simulink library "WZM_QSS_Lib"  (Simulink 7.7)
settings: Solver=ode45  StartTime=0.0  StopTime=10.0  RelTol=1e-3
undefined symbols (not defined in the file): A, AirCompressor, CNC, Housing, HydraulicPump, MainDrive, MainDriveCoolingEx, Process, ProcessCooling, R
libraries: WZM_QSS_Lib x36
(part 1 of 2)
settings Model: Creator=simon  LastModifiedBy=Coni

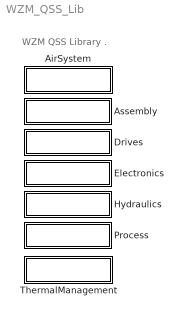
== system WZM_QSS_Lib ==
  note: WZM QSS Library
      | .
  AirSystem : Subsystem
      mask Display: disp('Air System')
  Assembly : Subsystem
      mask Display: disp('Assembly')
  Drives : Subsystem
      mask Display: disp('Drives')
  Electronics : Subsystem
      mask Display: disp('Electronics')
  Hydraulics : Subsystem
      mask Display: disp('Hydraulics')
  Process : Subsystem
      mask Display: disp('Process')
  ThermalManagement : Subsystem
      mask Display: disp('Thermal\nManagement')

== system WZM_QSS_Lib/AirSystem ==
  AirCompressor : Subsystem  BlockChoice=AirCompressor_Dummy
      settings: TemplateBlock=self  MemberBlocks=AirCompressor_Dummy,AirCompressor_Simple
  AirCompressor_Dummy : Subsystem
  AirCompressor_Simple : Subsystem  mask{Pstandby=0, Pworking=0}
      mask prompts: Pstandby "Standby consumption [W]"; Pworking "Working consumption [W]"

== system WZM_QSS_Lib/Assembly ==
  Turning Machine : Subsystem  mask{MainDrive=MainDrive, MainDriveCoolingEx=MainDriveCoolingEx, CNC=CNC, Process=Process, ProcessCooling=ProcessCooling, Housing=Housing, AirCompressor=AirCompressor, HydraulicPump=HydraulicPump, LocMainDrive=machine housing, LocProcessCooling=shop floor, LocProcess=process housing, LocMachine=shop floor, LocMachineExtr=shop floor, LocCNC=shop floor, LocCNCExtr=shop floor, LocAirCompressor=shop floor, LocHydraulicPump=shop floor}
      mask prompts: MainDrive "Main drive parameters"; MainDriveCoolingEx "Main drive cooling parameters"; CNC "CNC cabinet parameters"; Process "Process parameters"; ProcessCooling "Process cooling Parameters"; Housing "Housing Parameters"; AirCompressor "Air compressor Parameters"; HydraulicPump "Hydraulic pump Parameters"; LocMainDrive "Main drive cooling heat flow to"; LocProcessCooling "Process cooling heat flow to"; LocProcess "Process heat flow to"; LocMachine "Machine convective heat flow to"; LocMachineExtr "Machine cooling heat flow to"; LocCNC "Cabinet convective heat flow to"; LocCNCExtr "Cabinet cooling heat flow to"; LocAirCompressor "Air compressor heat flow to"; LocHydraulicPump "Hydraulic pump heat flow to"
      mask help:
      | Simple turning machine with:
      | - Air cooled process
      | - Air cooled machine housing
      | - Air-ar cooled cabinet
      mask StyleString: edit,edit,edit,edit,edit,edit,edit,edit,popup(process housing|machine housing|shop floor|external cooling),popup(process housing|machine housing|shop floor|external cooling),popup(process housing|machine housing|shop floor|external cooling),popup(process housing|machine housing|shop floor|external cooling),popup(process housing|machine housing|shop floor|external cooling),popup(process housing|machine housing|shop floor|external cooling),popup(process housing|machine housing|shop floor|external cooling),popup(process housing|machine housing|shop floor|external cooling),popup(process housing|machine housing|shop floor|external cooling)
      mask TabNameString: Parameters,Parameters,Parameters,Parameters,Parameters,Parameters,Parameters,Parameters,Heat management,Heat management,Heat management,Heat management,Heat management,Heat management,Heat management,Heat management,Heat management

== system WZM_QSS_Lib/Drives ==
  MainDrive : Subsystem  BlockChoice=MainDrive_simple
      settings: TemplateBlock=self  MemberBlocks=MainDrive_Dummy,MainDrive_simple
  MainDrive_Dummy : Subsystem  mask{P_max=20e3, eta=0.92, theta=1}
      mask prompts: P_max "Maximal mechanical power [W]"; eta "Efficiency of the motor [1]"; theta "Momentum of inertia of the drive [kg m^2]"
      mask help: Maps a demanded rotational speed and torque to the corresponding energy demand, heat generation and avaiable mechanical power.
      mask Display: disp('MAIN DRIVE');
  MainDrive_simple : Subsystem  mask{P_max=20e3, eta=0.92, theta=1, Tomega=MainDrive.Tabelomega, TM=MainDrive.TabelM, Teta=MainDrive.Tabeleta}
      mask prompts: P_max "Maximal mechanical power [W]"; eta "Efficiency of the motor [1]"; theta "Momentum of inertia of the drive [kg m^2]"; Tomega "Tabel omega"; TM "Tabel M"; Teta "Teabel eta"
      mask help: Maps a demanded rotational speed and torque to the corresponding energy demand, heat generation and avaiable mechanical power.
      mask Display: disp('MAIN DRIVE');
  Motor : Subsystem  mask{Pmax=10000, eta=.9, g=on}
      mask prompts: Pmax "Maximal absolute mechanical power [W]"; eta "Efficiency [1]"; g "Generator mode possible"
      mask help: Simple motor model. Maps the input u=P_dem/P_max to the produced mechanical power, the generated heat and the demanded electrical power.

== system WZM_QSS_Lib/Electronics ==
  CNC_Cabinet : Subsystem  BlockChoice=CNC_Cabinet_AirCooledFan_ao
      settings: TemplateBlock=self  MemberBlocks=CNC_Cabinet_AirAirCooled_Hyst,CNC_Cabinet_AirCooledFan_ao
  CNC_Cabinet_AirAirCooled_Hyst : Subsystem  mask{Cabinet=0, Cooling=0, SimoDrive=0}
      mask prompts: Cabinet "Cabinet Parameters"; Cooling "Air-air-cooling Parameters"; SimoDrive "Simodrive Parameters"
      mask help:
      | Parameters:
      |
      | - Cabinet.m
      | - Cabinet.cp
      | - Cabinet.R
      | - Cabinet.A
      |
      | - SimoDrive.OpPointsP
      | - SimoDrive.OpPointsEta
      | - SimoDrive.PStandby
      |
      | - Cooling.T_int
      | - Cooling.T_ext
      | - Cooling.Qdot
      | - Cooling.Tmin
      | - Cooling.Tmax
  CNC_Cabinet_AirCooledFan_ao : Subsystem  mask{Cabinet=0, Fan=0, SimoDrive=0}
      mask prompts: Cabinet "Cabinet Parameters"; Fan "Fan Parameters"; SimoDrive "Simodrive Parameters"
      mask help:
      | Parameters:
      |
      | - Cabinet.m
      | - Cabinet.cp
      | - Cabinet.R
      | - Cabinet.A
      |
      | - SimoDrive.OpPointsP
      | - SimoDrive.OpPointsEta
      | - SimoDrive.PStandby
      |
      | - Fan.Vdotnom
      | - Fan.Pnom
  Simodrive : Subsystem  mask{OpPointsP=0, OpPointsEta=0, Pstandby=0, g=off}
      mask prompts: OpPointsP "Operation points [W]"; OpPointsEta "Corresponding efficiencies [-]"; Pstandby "Standby consumption [W]"; g "Enable negative power"
      mask init:
      | if g==1
      |     g=-inf;
      | end

== system WZM_QSS_Lib/Hydraulics ==
  HydraulicPump : Subsystem  BlockChoice=HydraulicPump_Dummy
      settings: TemplateBlock=self  MemberBlocks=HydraulicPump_Dummy,HydraulicPump_Simple
  HydraulicPump_Dummy : Subsystem
  HydraulicPump_Simple : Subsystem  mask{Pconst=0}
      mask prompts: Pconst "Power consumption when running [W]"

== system WZM_QSS_Lib/Process ==
  ProcessModel : Subsystem  BlockChoice=Process_simple
      settings: TemplateBlock=self  MemberBlocks=Process_dummy,Process_simple
  Process_dummy : Subsystem
  Process_simple : Subsystem  mask{eta=0}
      mask prompts: eta "Efficiency of the process [1]"
      mask help: Simple process model: Mechanical work is converted to process work with constant efficiency

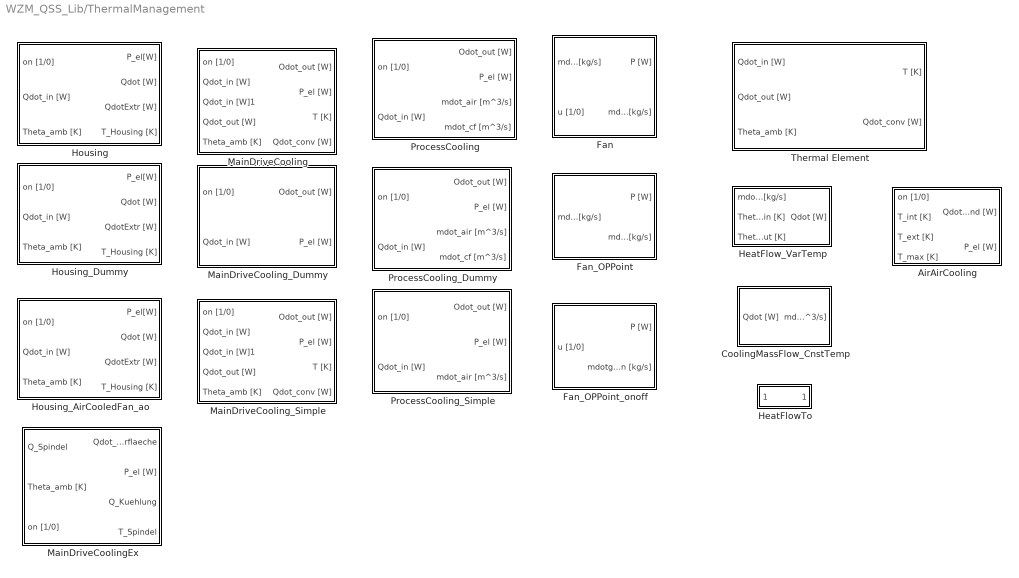
== system WZM_QSS_Lib/ThermalManagement ==
  AirAirCooling : Subsystem  mask{T_int_Pnts=0, T_amb_Pnts=0, Qdot_extr_Pnts=0, epsilon=0}
      mask prompts: T_int_Pnts "Internal temperature operation points [K]"; T_amb_Pnts "External temperature operation points [K]"; Qdot_extr_Pnts "Corresponding heat flow f(T_int,T_ext) [W]"; epsilon "COP of the cooling element"
  CoolingMassFlow_CnstTemp : Subsystem  mask{cp=0, Tin=0, Tout=0}
      mask prompts: cp "Internal heat capacity of the medium [J/kg/k]"; Tin "Inlet temperature [K]"; Tout "Outlet temperature [K]"
  Fan : Subsystem  BlockChoice=Fan_OPPoint
      settings: TemplateBlock=self  MemberBlocks=Fan_OPPoint,Fan_OPPoint_onoff
  Fan_OPPoint : Subsystem  mask{Vdotnom=1, Pnom=1, rho=1.2}
      mask prompts: Vdotnom "Nominal troughput [m^3/s]"; Pnom "Nominal electrical power consumption [W]"; rho "Desity of the  [kg/m^3]"
      mask help:
      | Simple model of a ventilator. Given a nominal operation point:
      | P = Pnom*(Vdem/Vnom)^3
      settings: AttributesFormatString=Vdotnom = %<Vdotnom> m^3/s\nPnom = %<Pnom> W\nDesity = %<rho> kg/m^3
      mask Display:
      | a = 0:.1:2*pi;
      | plot(.5+.3*cos(a),.5+.3*sin(a))
      | a1 = pi/6;
      | a2 = pi/2+pi/6;
      | x = .5+.3*[cos(a1), cos(a2)];
      | y = .5+.3*[sin(a1), sin(a2)];
      | plot(x,y)
      | plot(x([2 1]),y-.4)
  Fan_OPPoint_onoff : Subsystem  mask{Vdotnom=1, Pnom=1, rho=1.2}
      mask prompts: Vdotnom "Nominal troughput [m^3/s]"; Pnom "Nominal electrical power consumption [W]"; rho "Desity of the  [kg/m^3]"
      mask help:
      | Simple model of a ventilator. Given a nominal operation point:
      | P = Pnom*(Vdem/Vnom)^3
      settings: AttributesFormatString=Vdotnom = %<Vdotnom> m^3/s\nPnom = %<Pnom> W\nDesity = %<rho> kg/m^3
      mask Display:
      | a = 0:.1:2*pi;
      | plot(.5+.3*cos(a),.5+.3*sin(a))
      | a1 = pi/6;
      | a2 = pi/2+pi/6;
      | x = .5+.3*[cos(a1), cos(a2)];
      | y = .5+.3*[sin(a1), sin(a2)];
      | plot(x,y)
      | plot(x([2 1]),y-.4)
  HeatFlowTo : Subsystem  mask{Loc=process housing, LocNum=0}
      mask prompts: Loc "Heat flow to"; LocNum "Heat flow to 1=process housing, 2=machine housing, 3=shop floor, 4=external cooling (Keep zero while using popup above)]"
      mask help: Defines where the heat flux is going to
      mask init:
      | if LocNum ~=0
      |     Loc = LocNum;
      | end
      | 
      | idx = zeros(4,1);
      | idx(Loc)=1;
      settings: AttributesFormatString=%<Loc>
      mask StyleString: popup(process housing|machine housing|shop floor|external cooling),edit
      mask TabNameString: Popup,Numeric
      mask Display:
      | plot([0 1],[0.5 .9])
      | plot([0 1],[0.5 .6])
      | plot([0 1],[0.5 .4])
      | plot([0 1],[0.5 .1])
      | plot([1 1],[1 0])
  HeatFlow_VarTemp : Subsystem  mask{cp=1200}
      mask prompts: cp "Internal heat capacity of the medium [J/kg/k]"
  Housing : Subsystem  BlockChoice=Housing_AirCooledFan_ao
      settings: TemplateBlock=self  MemberBlocks=Housing_AirCooledFan_ao,Housing_Dummy
  Housing_AirCooledFan_ao : Subsystem  mask{Cabinet=0, Fan=0}
      mask prompts: Cabinet "Housing Parameters"; Fan "Fan Parameters"
      mask help:
      | Parameters:
      |
      | - Cabinet.m
      | - Cabinet.cp
      | - Cabinet.R
      | - Cabinet.A
      |
      | - Fan.Vdotnom
      | - Fan.Pnom
  Housing_Dummy : Subsystem
  MainDriveCooling : Subsystem  BlockChoice=MainDriveCooling_Dummy
      settings: TemplateBlock=self  MemberBlocks=MainDriveCooling_Dummy,MainDriveCooling_Simple
  MainDriveCoolingEx : Subsystem  mask{Temperatur=MainDriveCoolingEx.Temperatur, AirCooling=MainDriveCoolingEx.Air, TController=MainDriveCoolingEx}
      mask prompts: Temperatur "Tempeatur"; TController "TemperaturController"
  MainDriveCooling_Dummy : Subsystem
  MainDriveCooling_Simple : Subsystem  mask{OpPointQ=0, OpPointEpsilon=0, Pon=0}
      mask prompts: OpPointQ "Operation point heat flow"; OpPointEpsilon "Corresponding cooling index"; Pon "Idle consumption [W]"
  ProcessCooling : Subsystem  BlockChoice=ProcessCooling_Dummy
      settings: TemplateBlock=self  MemberBlocks=ProcessCooling_Dummy,ProcessCooling_Simple
  ProcessCooling_Dummy : Subsystem
  ProcessCooling_Simple : Subsystem  mask{Pconst=0}
      mask prompts: Pconst "Constant power demand [W]"
  Thermal Element : Subsystem  mask{m=10, cp=1200, R=0, A=2}
      mask prompts: m "Internal mass [kg]"; cp "Internal heat capacity [J/kg/K]"; R "Heat transfer resistance of the surface [W/m^2/K]"; A "Surface area [m^2]"
      mask help: Simple

== system WZM_QSS_Lib/AirSystem/AirCompressor ==
  on [1/0] : Inport
  mdot [kg/s] : Inport  Port=2
  AirCompressor_Dummy : WZM_QSS_Lib/AirSystem/AirCompressor_Dummy  SystemSampleTime=-1
  P_el [W] : Outport
  Qdot [W] : Outport  Port=2
  wires:
  on [1/0]/1 -> AirCompressor_Dummy/1
  mdot [kg/s]/1 -> AirCompressor_Dummy/2
  AirCompressor_Dummy/1 -> P_el [W]/1
  AirCompressor_Dummy/2 -> Qdot [W]/1

== system WZM_QSS_Lib/AirSystem/AirCompressor_Dummy ==
  on [1/0] : Inport
  mdot [kg/s] : Inport  Port=2
  Constant : Constant  Value=0
  Constant1 : Constant  Value=0
  Terminator : Terminator
  Terminator1 : Terminator
  P_el [W] : Outport
  Qdot [W] : Outport  Port=2
  wires:
  Constant/1 -> P_el [W]/1
  Constant1/1 -> Qdot [W]/1
  on [1/0]/1 -> Terminator/1
  mdot [kg/s]/1 -> Terminator1/1

== system WZM_QSS_Lib/AirSystem/AirCompressor_Simple ==
  on [1/0] : Inport
  mdot [kg/s] : Inport  Port=2
  Constant : Constant  Value=0
  Constant1 : Constant  Value=Pstandby
  Constant2 : Constant  Value=Pworking
  Switch : Switch  Criteria=u2 > Threshold
  Switch1 : Switch  Criteria=u2 > Threshold
  P_el [W] : Outport
  wires:
  Switch/1 -> P_el [W]/1
  on [1/0]/1 -> Switch/2
  mdot [kg/s]/1 -> Switch1/2
  Switch1/1 -> Switch/1
  Constant2/1 -> Switch1/1
  Constant/1 -> Switch1/3
  Constant1/1 -> Switch/3

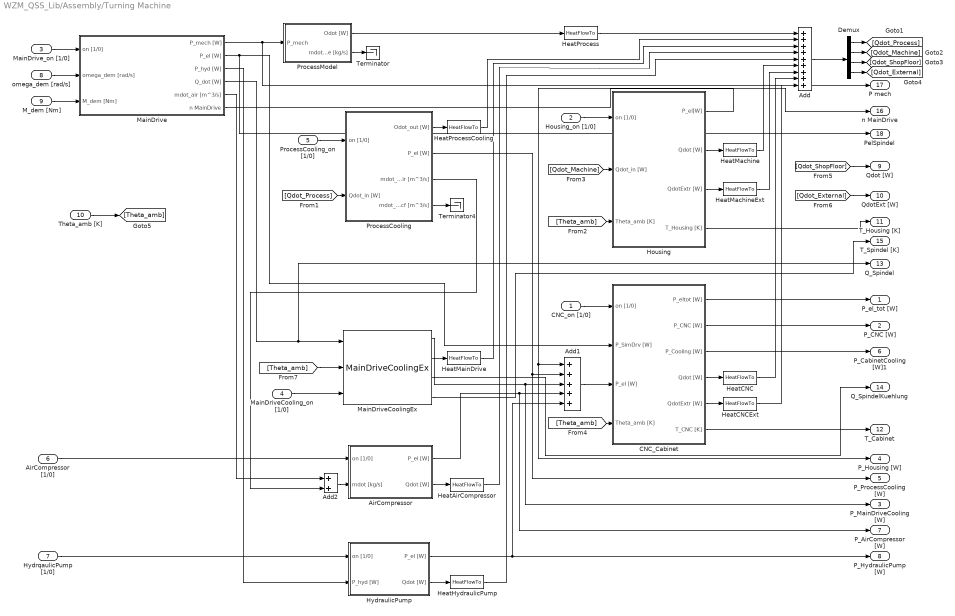
== system WZM_QSS_Lib/Assembly/Turning Machine ==
  CNC_on [1/0] : Inport
  Housing_on [1/0] : Inport  Port=2
  MainDrive_on [1/0] : Inport  Port=3
  MainDriveCooling_on [1/0] : Inport  Port=4
  ProcessCooling_on [1/0] : Inport  Port=5
  AirCompressor [1/0] : Inport  Port=6
  HydrqaulicPump [1/0] : Inport  Port=7
  omega_dem [rad/s] : Inport  Port=8
  M_dem [Nm] : Inport  Port=9
  Theta_amb [K] : Inport  Port=10
  Add : Sum  Inputs=+++++++++
  Add1 : Sum  Inputs=+++++
  Add2 : Sum
  AirCompressor : Subsystem  BlockChoice=AirCompressor_Simple
      link override AirCompressor_Simple: Pstandby=AirCompressor.Pstandby  Pworking=AirCompressor.Pworking
      settings: AttributesFormatString=%<BlockChoice>  TemplateBlock=WZM_QSS_Lib/AirSystem/AirCompressor  MemberBlocks=AirCompressor_Dummy,AirCompressor_Simple
  CNC_Cabinet : Subsystem  BlockChoice=CNC_Cabinet_AirAirCooled_Hyst
      link override CNC_Cabinet_AirAirCooled_Hyst: Cabinet=CNC.Cabinet  Cooling=CNC.Cooling  SimoDrive=CNC.SimoDrive
      link override CNC_Cabinet_AirCooledFan_ao: Cabinet=CNC.Cabinet  Fan=CNC.Fan  PstandbySDSimoDrive=CNC.Fan  SimoDrive=CNC.SimoDrive
      settings: AttributesFormatString=%<BlockChoice>  TemplateBlock=WZM_QSS_Lib/Electronics/CNC_Cabinet  MemberBlocks=CNC_Cabinet_AirAirCooled_Hyst,CNC_Cabinet_AirCooledFan_ao
  Demux : Demux
  HeatAirCompressor : WZM_QSS_Lib/ThermalManagement/HeatFlowTo  SystemSampleTime=-1  Loc=machine housing  LocNum=LocAirCompressor
      settings: AttributesFormatString=%<Loc>
  HeatCNC : WZM_QSS_Lib/ThermalManagement/HeatFlowTo  SystemSampleTime=-1  Loc=shop floor  LocNum=LocCNC
      settings: AttributesFormatString=%<Loc>
  HeatCNCExt : WZM_QSS_Lib/ThermalManagement/HeatFlowTo  SystemSampleTime=-1  Loc=shop floor  LocNum=LocCNCExtr
      settings: AttributesFormatString=%<Loc>
  HeatHydraulicPump : WZM_QSS_Lib/ThermalManagement/HeatFlowTo  SystemSampleTime=-1  Loc=machine housing  LocNum=LocHydraulicPump
      settings: AttributesFormatString=%<Loc>
  HeatMachine : WZM_QSS_Lib/ThermalManagement/HeatFlowTo  SystemSampleTime=-1  Loc=shop floor  LocNum=LocMachine
      settings: AttributesFormatString=%<Loc>
  HeatMachineExt : WZM_QSS_Lib/ThermalManagement/HeatFlowTo  SystemSampleTime=-1  Loc=shop floor  LocNum=LocMachineExtr
      settings: AttributesFormatString=%<Loc>
  HeatMainDrive : WZM_QSS_Lib/ThermalManagement/HeatFlowTo  SystemSampleTime=-1  Loc=machine housing  LocNum=LocMainDrive
      settings: AttributesFormatString=%<Loc>
  HeatProcess : WZM_QSS_Lib/ThermalManagement/HeatFlowTo  SystemSampleTime=-1  Loc=process housing  LocNum=LocProcess
      settings: AttributesFormatString=%<Loc>
  HeatProcessCooling : WZM_QSS_Lib/ThermalManagement/HeatFlowTo  SystemSampleTime=-1  Loc=shop floor  LocNum=LocProcessCooling
      settings: AttributesFormatString=%<Loc>
  Housing : Subsystem  BlockChoice=Housing_AirCooledFan_ao
      link override Housing_AirCooledFan_ao: Cabinet=Housing.Cabinet  Fan=Housing.Fan
      settings: AttributesFormatString=%<BlockChoice>  TemplateBlock=WZM_QSS_Lib/ThermalManagement/Housing  MemberBlocks=Housing_AirCooledFan_ao,Housing_Dummy
  HydraulicPump : Subsystem  BlockChoice=HydraulicPump_Simple
      link override HydraulicPump_Simple: Pconst=HydraulicPump.Pconst
      settings: AttributesFormatString=%<BlockChoice>  TemplateBlock=WZM_QSS_Lib/Hydraulics/HydraulicPump  MemberBlocks=HydraulicPump_Dummy,HydraulicPump_Simple
  MainDrive : Subsystem  BlockChoice=MainDrive_simple
      link override MainDrive_simple: P_max=MainDrive.Pmax  eta=MainDrive.eta  theta=MainDrive.Theta
      settings: AttributesFormatString=%<BlockChoice>  TemplateBlock=WZM_QSS_Lib/Drives/MainDrive  MemberBlocks=MainDrive_Dummy,MainDrive_simple
  MainDriveCoolingEx : WZM_QSS_Lib/ThermalManagement/MainDriveCoolingEx  SystemSampleTime=-1  Temperatur=MainDriveCoolingEx.Temperatur  AirCooling=MainDriveCoolingEx.Air  TController=MainDriveCoolingEx
  ProcessCooling : Subsystem  BlockChoice=ProcessCooling_Simple
      link override ProcessCooling_Simple: Pconst=ProcessCooling.Pconst
      settings: AttributesFormatString=%<BlockChoice>  TemplateBlock=WZM_QSS_Lib/ThermalManagement/ProcessCooling  MemberBlocks=ProcessCooling_Dummy,ProcessCooling_Simple
  ProcessModel : Subsystem  BlockChoice=Process_simple
      link override Process_simple: eta=Process.eta
      settings: AttributesFormatString=%<BlockChoice>  TemplateBlock=WZM_QSS_Lib/Process/ProcessModel  MemberBlocks=Process_dummy,Process_simple
  Terminator : Terminator
  Terminator4 : Terminator
  P_el_tot [W] : Outport
  P_CNC [W] : Outport  Port=2
  P_MainDriveCooling [W] : Outport  Port=3
  P_Housing [W] : Outport  Port=4
  P_ProcessCooling [W] : Outport  Port=5
  P_CabinetCooling [W]1 : Outport  Port=6
  P_AirCompressor [W] : Outport  Port=7
  P_HydraulicPump [W] : Outport  Port=8
  Qdot [W] : Outport  Port=9
  QdotExt [W] : Outport  Port=10
  T_Housing [K] : Outport  Port=11
  T_Cabinet : Outport  Port=12
  Q_Spindel : Outport  Port=13
  Q_SpindelKuehlung : Outport  Port=14
  T_Spindel [K] : Outport  Port=15
  n MainDrive : Outport  Port=16
  P mech : Outport  Port=17
  PelSpindel : Outport  Port=18
  wires:
  MainDriveCooling_on [1/0]/1 -> MainDriveCoolingEx/3
  [Theta_amb] -> MainDriveCoolingEx/2
  MainDrive/1(P_mech [W]) -> ProcessModel/1(P_mech), P mech/1
  CNC_Cabinet/1(P_eltot [W]) -> P_el_tot [W]/1
  CNC_on [1/0]/1 -> CNC_Cabinet/1(on [1/0])
  ProcessModel/1(Odot [W]) -> HeatProcess/1
  Add/1 -> Demux/1
  Demux/1 -> [Qdot_Process]
  Demux/2 -> [Qdot_Machine]
  Demux/3 -> [Qdot_ShopFloor]
  Demux/4 -> [Qdot_External]
  HeatProcess/1 -> Add/1
  HeatCNC/1 -> Add/8
  HeatCNCExt/1 -> Add/9
  Housing_on [1/0]/1 -> Housing/1(on [1/0])
  Theta_amb [K]/1 -> [Theta_amb]
  [Theta_amb] -> Housing/3(Theta_amb [K])
  [Qdot_Machine] -> Housing/2(Qdot_in [W])
  [Theta_amb] -> CNC_Cabinet/4(Theta_amb [K])
  Housing/2(Qdot [W]) -> HeatMachine/1
  Housing/3(QdotExtr [W]) -> HeatMachineExt/1
  HeatMachineExt/1 -> Add/7
  HeatMachine/1 -> Add/6
  Add1/1 -> CNC_Cabinet/3(P_el [W])
  Housing/1(P_el[W]) -> Add1/1, P_Housing [W]/1
  [Qdot_ShopFloor] -> Qdot [W]/1
  [Qdot_External] -> QdotExt [W]/1
  Housing/4(T_Housing [K]) -> T_Housing [K]/1
  MainDriveCoolingEx/2 -> Add1/3, P_MainDriveCooling [W]/1
  MainDriveCoolingEx/1 -> HeatMainDrive/1
  ProcessModel/2(mdot_waste [kg/s]) -> Terminator/1
  M_dem [Nm]/1 -> MainDrive/3(M_dem [Nm])
  omega_dem [rad/s]/1 -> MainDrive/2(omega_dem [rad/s])
  MainDrive_on [1/0]/1 -> MainDrive/1(on [1/0])
  ProcessCooling_on [1/0]/1 -> ProcessCooling/1(on [1/0])
  [Qdot_Process] -> ProcessCooling/2(Qdot_in [W])
  MainDrive/3(P_hyd [W]) -> HydraulicPump/2(P_hyd [W])
  MainDrive/2(P_el [W]) -> CNC_Cabinet/2(P_SimDrv [W]), PelSpindel/1
  ProcessCooling/1(Odot_out [W]) -> HeatProcessCooling/1
  HeatMainDrive/1 -> Add/3
  HeatProcessCooling/1 -> Add/2
  ProcessCooling/2(P_el [W]) -> Add1/2, P_ProcessCooling [W]/1
  ProcessCooling/3(mdot_air [m^3/s]) -> Add2/2
  ProcessCooling/4(mdot_cf [m^3/s]) -> Terminator4/1
  MainDrive/4(Q_dot [W]) -> MainDriveCoolingEx/1, Q_Spindel/1
  CNC_Cabinet/2(P_CNC [W]) -> P_CNC [W]/1
  CNC_Cabinet/6(T_CNC [K]) -> T_Cabinet/1
  CNC_Cabinet/5(QdotExtr [W]) -> HeatCNCExt/1
  CNC_Cabinet/4(Qdot [W]) -> HeatCNC/1
  CNC_Cabinet/3(P_Cooling [W]) -> P_CabinetCooling [W]1/1
  AirCompressor/1(P_el [W]) -> Add1/4, P_AirCompressor [W]/1
  AirCompressor/2(Qdot [W]) -> HeatAirCompressor/1
  HeatAirCompressor/1 -> Add/4
  Add2/1 -> AirCompressor/2(mdot [kg/s])
  MainDrive/5(mdot_air [m^3/s]) -> Add2/1
  AirCompressor [1/0]/1 -> AirCompressor/1(on [1/0])
  HydraulicPump/1(P_el [W]) -> Add1/5, P_HydraulicPump [W]/1
  HydrqaulicPump [1/0]/1 -> HydraulicPump/1(on [1/0])
  HydraulicPump/2(Qdot [W]) -> HeatHydraulicPump/1
  HeatHydraulicPump/1 -> Add/5
  MainDriveCoolingEx/3 -> Q_SpindelKuehlung/1
  MainDriveCoolingEx/4 -> T_Spindel [K]/1
  MainDrive/6(n MainDrive) -> n MainDrive/1

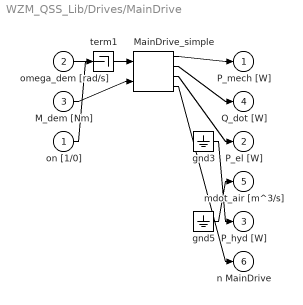
== system WZM_QSS_Lib/Drives/MainDrive ==
  on [1/0] : Inport
  omega_dem [rad/s] : Inport  Port=2
  M_dem [Nm] : Inport  Port=3
  MainDrive_simple : WZM_QSS_Lib/Drives/MainDrive_simple  SystemSampleTime=-1  P_max=20e3  eta=0.92  theta=1  Tomega=MainDrive.Tabelomega  TM=MainDrive.TabelM  Teta=MainDrive.Tabeleta
  gnd3 : Ground
  gnd5 : Ground
  term1 : Terminator
  P_mech [W] : Outport
  P_el [W] : Outport  Port=2
  P_hyd [W] : Outport  Port=3
  Q_dot [W] : Outport  Port=4
  mdot_air [m^3/s] : Outport  Port=5
  n MainDrive : Outport  Port=6
  wires:
  omega_dem [rad/s]/1 -> MainDrive_simple/1
  M_dem [Nm]/1 -> MainDrive_simple/2
  MainDrive_simple/1 -> P_mech [W]/1
  MainDrive_simple/2 -> Q_dot [W]/1
  MainDrive_simple/3 -> P_el [W]/1
  MainDrive_simple/4 -> n MainDrive/1
  on [1/0]/1 -> term1/1
  gnd3/1 -> P_hyd [W]/1
  gnd5/1 -> mdot_air [m^3/s]/1

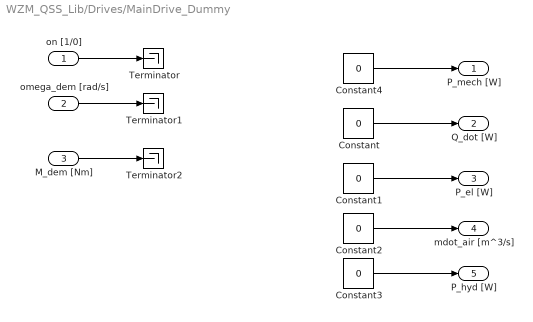
== system WZM_QSS_Lib/Drives/MainDrive_Dummy ==
  on [1/0] : Inport
  omega_dem [rad/s] : Inport  Port=2
  M_dem [Nm] : Inport  Port=3
  Constant{,1..4} (5 alike) : Constant  Value=0
  Terminator : Terminator
  Terminator1 : Terminator
  Terminator2 : Terminator
  P_mech [W] : Outport
  Q_dot [W] : Outport  Port=2
  P_el [W] : Outport  Port=3
  mdot_air [m^3/s] : Outport  Port=4
  P_hyd [W] : Outport  Port=5
  wires:
  on [1/0]/1 -> Terminator/1
  omega_dem [rad/s]/1 -> Terminator1/1
  M_dem [Nm]/1 -> Terminator2/1
  Constant4/1 -> P_mech [W]/1
  Constant/1 -> Q_dot [W]/1
  Constant1/1 -> P_el [W]/1
  Constant2/1 -> mdot_air [m^3/s]/1
  Constant3/1 -> P_hyd [W]/1

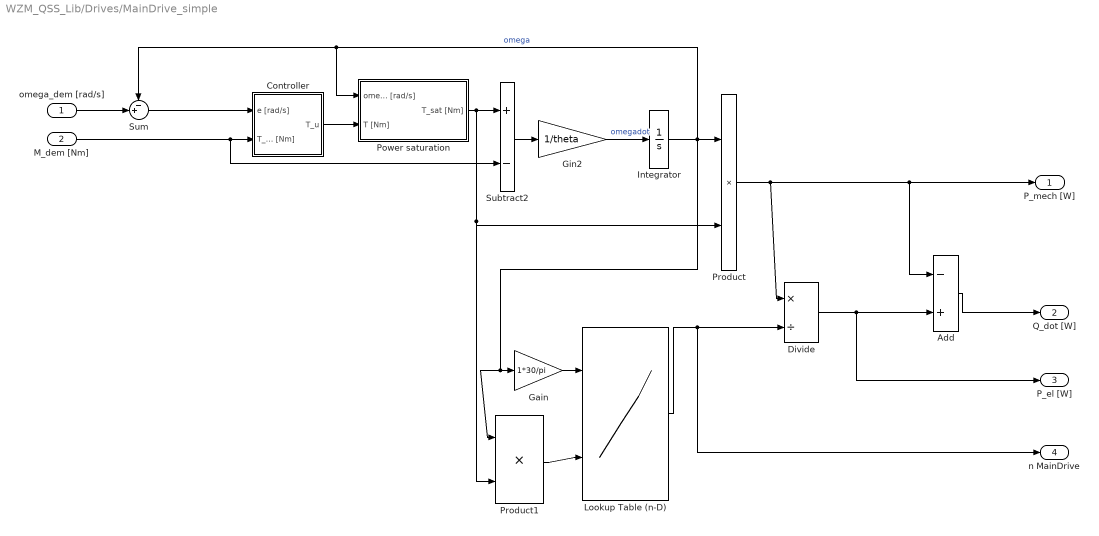
== system WZM_QSS_Lib/Drives/MainDrive_simple ==
  omega_dem [rad/s] : Inport
  M_dem [Nm] : Inport  Port=2
  Add : Sum  Inputs=-+
  Controller : Subsystem
  Divide : Product  Inputs=*/
  Gain : Gain  Gain=1*30/pi
  Gin2 : Gain  Gain=1/theta
  Integrator : Integrator
  Lookup Table (n-D) : Lookup_n-D  BreakpointsForDimension1=Tomega  BreakpointsForDimension2=TM  Table=Teta  InterpMethod=Cubic spline  ExtrapMethod=Cubic spline  InputSameDT=on
  Power saturation : Subsystem
  Product : Product  RndMeth=Zero
  Product1 : Product  RndMeth=Zero
  Subtract2 : Sum  Inputs=+-
  Sum : Sum  Inputs=-+|
  P_mech [W] : Outport
  Q_dot [W] : Outport  Port=2
  P_el [W] : Outport  Port=3
  n MainDrive : Outport  Port=4
  wires:
  Integrator/1 -> Product/1, Sum/1, Power saturation/1(omega [rad/s]), Gain/1, Product1/1  "omega"
  Product/1 -> Divide/1, P_mech [W]/1, Add/1
  Gin2/1 -> Integrator/1  "omegadot"
  omega_dem [rad/s]/1 -> Sum/2
  Sum/1 -> Controller/1(e [rad/s])
  M_dem [Nm]/1 -> Subtract2/2, Controller/2(T_dem [Nm])
  Controller/1(T_u) -> Power saturation/2(T [Nm])
  Subtract2/1 -> Gin2/1
  Power saturation/1(T_sat [Nm]) -> Subtract2/1, Product/2, Product1/2
  Add/1 -> Q_dot [W]/1
  Lookup Table (n-D)/1 -> Divide/2, n MainDrive/1
  Divide/1 -> P_el [W]/1, Add/2
  Gain/1 -> Lookup Table (n-D)/1
  Product1/1 -> Lookup Table (n-D)/2

== system WZM_QSS_Lib/Drives/Motor ==
  u [1] : Inport
  Abs : Abs
  Saturation : Saturate  UpperLimit=1  LowerLimit=-g
  ain : Gain  Gain=Pmax
  ain1 : Gain  Gain=1/eta-1
  ain2 : Gain  Gain=1/eta
  P_mech [W] : Outport
  Qdot [W] : Outport  Port=2
  P_el [W] : Outport  Port=3
  wires:
  u [1]/1 -> Saturation/1
  Saturation/1 -> ain/1
  ain/1 -> P_mech [W]/1, ain2/1, Abs/1
  ain1/1 -> Qdot [W]/1
  ain2/1 -> P_el [W]/1
  Abs/1 -> ain1/1

== system WZM_QSS_Lib/Electronics/CNC_Cabinet ==
  on [1/0] : Inport
  P_SimDrv [W] : Inport  Port=2
  P_el [W] : Inport  Port=3
  Theta_amb [K] : Inport  Port=4
  CNC_Cabinet_AirCooledFan_ao : WZM_QSS_Lib/Electronics/CNC_Cabinet_AirCooledFan_ao  SystemSampleTime=-1  Cabinet=0  Fan=0  SimoDrive=0
  gnd3 : Ground
  P_eltot [W] : Outport
  P_CNC [W] : Outport  Port=2
  P_Cooling [W] : Outport  Port=3
  Qdot [W] : Outport  Port=4
  QdotExtr [W] : Outport  Port=5
  T_CNC [K] : Outport  Port=6
  wires:
  on [1/0]/1 -> CNC_Cabinet_AirCooledFan_ao/1
  P_SimDrv [W]/1 -> CNC_Cabinet_AirCooledFan_ao/2
  P_el [W]/1 -> CNC_Cabinet_AirCooledFan_ao/3
  Theta_amb [K]/1 -> CNC_Cabinet_AirCooledFan_ao/4
  CNC_Cabinet_AirCooledFan_ao/1 -> P_eltot [W]/1
  CNC_Cabinet_AirCooledFan_ao/2 -> P_CNC [W]/1
  CNC_Cabinet_AirCooledFan_ao/3 -> Qdot [W]/1
  CNC_Cabinet_AirCooledFan_ao/4 -> QdotExtr [W]/1
  CNC_Cabinet_AirCooledFan_ao/5 -> T_CNC [K]/1
  gnd3/1 -> P_Cooling [W]/1

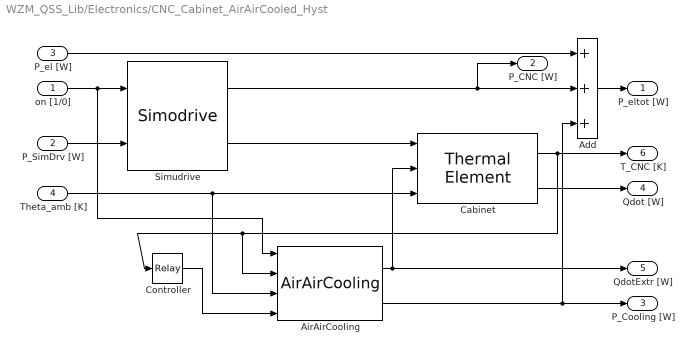
== system WZM_QSS_Lib/Electronics/CNC_Cabinet_AirAirCooled_Hyst ==
  on [1/0] : Inport
  P_SimDrv [W] : Inport  Port=2
  P_el [W] : Inport  Port=3
  Theta_amb [K] : Inport  Port=4
  Add : Sum  Inputs=+++
  AirAirCooling : WZM_QSS_Lib/ThermalManagement/AirAirCooling  SystemSampleTime=-1  T_int_Pnts=Cooling.T_int  T_amb_Pnts=Cooling.T_ext  Qdot_extr_Pnts=Cooling.Qdot  epsilon=Cooling.epsilon
  Cabinet : WZM_QSS_Lib/ThermalManagement/Thermal Element  SystemSampleTime=-1  m=Cabinet.m  cp=Cabinet.cp  R=Cabinet.R  A=Cabinet.A
  Controller : Relay  OnSwitchValue=Cooling.Tmax  OffSwitchValue=Cooling.Tmin
  Simudrive : WZM_QSS_Lib/Electronics/Simodrive  SystemSampleTime=-1  OpPointsP=SimoDrive.OpPointsP  OpPointsEta=SimoDrive.OpPointsEta  Pstandby=SimoDrive.PStandby  g=off
  P_eltot [W] : Outport
  P_CNC [W] : Outport  Port=2
  P_Cooling [W] : Outport  Port=3
  Qdot [W] : Outport  Port=4
  QdotExtr [W] : Outport  Port=5
  T_CNC [K] : Outport  Port=6
  wires:
  on [1/0]/1 -> Simudrive/1, AirAirCooling/1
  Theta_amb [K]/1 -> Cabinet/3, AirAirCooling/3
  Cabinet/1 -> T_CNC [K]/1, Controller/1, AirAirCooling/2
  Add/1 -> P_eltot [W]/1
  Cabinet/2 -> Qdot [W]/1
  P_SimDrv [W]/1 -> Simudrive/2
  Simudrive/2 -> Cabinet/1
  Simudrive/1 -> P_CNC [W]/1, Add/2
  P_el [W]/1 -> Add/1
  AirAirCooling/1 -> QdotExtr [W]/1, Cabinet/2
  AirAirCooling/2 -> Add/3, P_Cooling [W]/1
  Controller/1 -> AirAirCooling/4

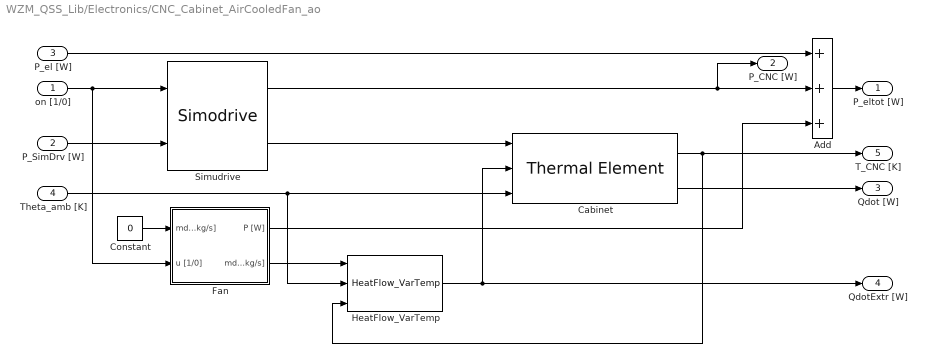
== system WZM_QSS_Lib/Electronics/CNC_Cabinet_AirCooledFan_ao ==
  on [1/0] : Inport
  P_SimDrv [W] : Inport  Port=2
  P_el [W] : Inport  Port=3
  Theta_amb [K] : Inport  Port=4
  Add : Sum  Inputs=+++
  Cabinet : WZM_QSS_Lib/ThermalManagement/Thermal Element  SystemSampleTime=-1  m=Cabinet.m  cp=Cabinet.cp  R=Cabinet.R  A=Cabinet.A
  Constant : Constant  Value=0
  Fan : Subsystem  BlockChoice=Fan_OPPoint_onoff
      link override Fan_OPPoint: Vdotnom=Fan.Vdotnom  Pnom=Fan.Pnom
      settings: AttributesFormatString=%<BlockChoice>  TemplateBlock=WZM_QSS_Lib/ThermalManagement/Fan  MemberBlocks=Fan_OPPoint,Fan_OPPoint_onoff
  HeatFlow_VarTemp : WZM_QSS_Lib/ThermalManagement/HeatFlow_VarTemp  SystemSampleTime=-1  cp=1005
  Simudrive : WZM_QSS_Lib/Electronics/Simodrive  SystemSampleTime=-1  OpPointsP=SimoDrive.OpPointsP  OpPointsEta=SimoDrive.OpPointsEta  Pstandby=SimoDrive.PStandby  g=off
  P_eltot [W] : Outport
  P_CNC [W] : Outport  Port=2
  Qdot [W] : Outport  Port=3
  QdotExtr [W] : Outport  Port=4
  T_CNC [K] : Outport  Port=5
  wires:
  P_el [W]/1 -> Add/1
  Simudrive/1 -> Add/2, P_CNC [W]/1
  Simudrive/2 -> Cabinet/1
  P_SimDrv [W]/1 -> Simudrive/2
  HeatFlow_VarTemp/1 -> QdotExtr [W]/1, Cabinet/2
  Fan/2(mdotgen [kg/s]) -> HeatFlow_VarTemp/1
  Cabinet/2 -> Qdot [W]/1
  Fan/1(P [W]) -> Add/3
  Add/1 -> P_eltot [W]/1
  Cabinet/1 -> HeatFlow_VarTemp/3, T_CNC [K]/1
  Theta_amb [K]/1 -> HeatFlow_VarTemp/2, Cabinet/3
  Constant/1 -> Fan/1(mdot [kg/s])
  on [1/0]/1 -> Simudrive/1, Fan/2(u [1/0])

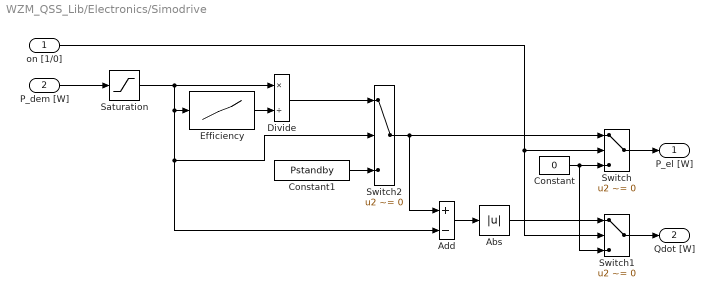
== system WZM_QSS_Lib/Electronics/Simodrive ==
  on [1/0] : Inport
  P_dem [W] : Inport  Port=2
  Abs : Abs
  Add : Sum  Inputs=+-
  Constant : Constant  Value=0
  Constant1 : Constant  Value=Pstandby
  Divide : Product  Inputs=*/
  Efficiency : Lookup_n-D  NumberOfTableDimensions=1  BreakpointsForDimension1=OpPointsP  Table=OpPointsEta  UseLastTableValue=on  RndMeth=Simplest  InputSameDT=on
  Saturation : Saturate  UpperLimit=Inf  LowerLimit=g
  Switch : Switch  Criteria=u2 ~= 0
  Switch1 : Switch  Criteria=u2 ~= 0
  Switch2 : Switch  Criteria=u2 ~= 0
  P_el [W] : Outport
  Qdot [W] : Outport  Port=2
  wires:
  Switch/1 -> P_el [W]/1
  Switch1/1 -> Qdot [W]/1
  Constant/1 -> Switch/3, Switch1/3
  P_dem [W]/1 -> Saturation/1
  Constant1/1 -> Switch2/3
  Efficiency/1 -> Divide/2
  on [1/0]/1 -> Switch1/2, Switch/2
  Add/1 -> Abs/1
  Switch2/1 -> Add/1, Switch/1
  Divide/1 -> Switch2/1
  Abs/1 -> Switch1/1
  Saturation/1 -> Divide/1, Efficiency/1, Switch2/2, Add/2

== system WZM_QSS_Lib/Hydraulics/HydraulicPump ==
  on [1/0] : Inport
  P_hyd [W] : Inport  Port=2
  HydraulicPump_Dummy : WZM_QSS_Lib/Hydraulics/HydraulicPump_Dummy  SystemSampleTime=-1
  P_el [W] : Outport
  Qdot [W] : Outport  Port=2
  wires:
  on [1/0]/1 -> HydraulicPump_Dummy/1
  P_hyd [W]/1 -> HydraulicPump_Dummy/2
  HydraulicPump_Dummy/1 -> P_el [W]/1
  HydraulicPump_Dummy/2 -> Qdot [W]/1

== system WZM_QSS_Lib/Hydraulics/HydraulicPump_Dummy ==
  on [1/0] : Inport
  P_hyd [W] : Inport  Port=2
  Constant : Constant  Value=0
  Constant1 : Constant  Value=0  LockScale=on
  Terminator : Terminator
  Terminator1 : Terminator
  P_el [W] : Outport
  Qdot [W] : Outport  Port=2
  wires:
  Constant/1 -> P_el [W]/1
  Constant1/1 -> Qdot [W]/1
  P_hyd [W]/1 -> Terminator/1
  on [1/0]/1 -> Terminator1/1

== system WZM_QSS_Lib/Hydraulics/HydraulicPump_Simple ==
  on [1/0] : Inport
  P_hyd [W] : Inport  Port=2
  Constant : Constant  Value=0
  Constant1 : Constant  Value=0  LockScale=on
  Constant2 : Constant  Value=Pconst
  Switch : Switch  Criteria=u2 > Threshold
  Terminator : Terminator
  P_el [W] : Outport
  Qdot [W] : Outport  Port=2
  wires:
  P_hyd [W]/1 -> Terminator/1
  Constant1/1 -> Qdot [W]/1
  Switch/1 -> P_el [W]/1
  on [1/0]/1 -> Switch/2
  Constant2/1 -> Switch/1
  Constant/1 -> Switch/3

== system WZM_QSS_Lib/Process/ProcessModel ==
  P_mech : Inport
  Process_simple : WZM_QSS_Lib/Process/Process_simple  SystemSampleTime=-1  eta=0
  gnd2 : Ground
  Odot [W] : Outport
  mdot_waste [kg/s] : Outport  Port=2
  wires:
  P_mech/1 -> Process_simple/1
  Process_simple/1 -> Odot [W]/1
  gnd2/1 -> mdot_waste [kg/s]/1

== system WZM_QSS_Lib/Process/Process_dummy ==
  P_mech : Inport
  Constant : Constant  Value=0
  Constant1 : Constant  Value=0
  Terminator : Terminator
  Odot [W] : Outport
  mdot_waste [kg/s] : Outport  Port=2
  wires:
  P_mech/1 -> Terminator/1
  Constant1/1 -> mdot_waste [kg/s]/1
  Constant/1 -> Odot [W]/1

== system WZM_QSS_Lib/Process/Process_simple ==
  P_mech : Inport
  Gain : Gain  Gain=1-eta
  Odot [W] : Outport
  wires:
  P_mech/1 -> Gain/1
  Gain/1 -> Odot [W]/1

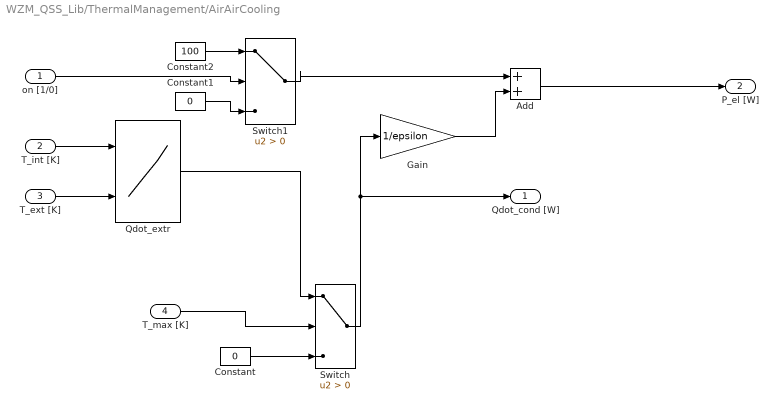
== system WZM_QSS_Lib/ThermalManagement/AirAirCooling ==
  on [1/0] : Inport
  T_int [K] : Inport  Port=2
  T_ext [K] : Inport  Port=3
  T_max [K] : Inport  Port=4
  Add : Sum
  Constant : Constant  Value=0
  Constant1 : Constant  Value=0
  Constant2 : Constant  Value=100
  Gain : Gain  Gain=1/epsilon
  Qdot_extr : Lookup_n-D  BreakpointsForDimension1=T_int_Pnts  BreakpointsForDimension2=T_amb_Pnts  Table=Qdot_extr_Pnts  InterpMethod=Cubic spline  RndMeth=Simplest  InputSameDT=on
  Switch : Switch  Criteria=u2 > Threshold
  Switch1 : Switch  Criteria=u2 > Threshold
  Qdot_cond [W] : Outport
  P_el [W] : Outport  Port=2
  wires:
  T_int [K]/1 -> Qdot_extr/1
  T_ext [K]/1 -> Qdot_extr/2
  Constant/1 -> Switch/3
  Qdot_extr/1 -> Switch/1
  Switch/1 -> Qdot_cond [W]/1, Gain/1
  on [1/0]/1 -> Switch1/2
  Constant1/1 -> Switch1/3
  Constant2/1 -> Switch1/1
  Switch1/1 -> Add/1
  Add/1 -> P_el [W]/1
  Gain/1 -> Add/2
  T_max [K]/1 -> Switch/2

== system WZM_QSS_Lib/ThermalManagement/CoolingMassFlow_CnstTemp ==
  Qdot [W] : Inport
  Gain : Gain  Gain=1/cp
  Gain1 : Gain  Gain=1/(Tout-Tin)
  mdot [m^3/s] : Outport
  wires:
  Qdot [W]/1 -> Gain/1
  Gain/1 -> Gain1/1
  Gain1/1 -> mdot [m^3/s]/1

== system WZM_QSS_Lib/ThermalManagement/Fan ==
  mdot [kg/s] : Inport
  u [1/0] : Inport  Port=2
  Fan_OPPoint : WZM_QSS_Lib/ThermalManagement/Fan_OPPoint  SystemSampleTime=-1  Vdotnom=1  Pnom=1  rho=1.2
      settings: AttributesFormatString=Vdotnom = %<Vdotnom> m^3/s\nPnom = %<Pnom> W\nDesity = %<rho> kg/m^3
  term2 : Terminator
  P [W] : Outport
  mdotgen [kg/s] : Outport  Port=2
  wires:
  mdot [kg/s]/1 -> Fan_OPPoint/1
  Fan_OPPoint/1 -> P [W]/1
  Fan_OPPoint/2 -> mdotgen [kg/s]/1
  u [1/0]/1 -> term2/1

== system WZM_QSS_Lib/ThermalManagement/Fan_OPPoint ==
  mdot [kg/s] : Inport
  Gain : Gain  Gain=1/rho/Vdotnom
  Gain1 : Gain  Gain=Pnom
  Product : Product  Inputs=3  RndMeth=Zero
  P [W] : Outport
  mdotgen [kg/s] : Outport  Port=2
  wires:
  mdot [kg/s]/1 -> Gain/1, mdotgen [kg/s]/1
  Gain/1 -> Product/1, Product/2, Product/3
  Product/1 -> Gain1/1
  Gain1/1 -> P [W]/1

== system WZM_QSS_Lib/ThermalManagement/Fan_OPPoint_onoff ==
  u [1/0] : Inport
  Constant : Constant
  Constant1 : Constant  Value=0
  Gain : Gain  Gain=rho*Vdotnom
  Gain1 : Gain  Gain=Pnom
  Switch : Switch  Criteria=u2 > Threshold
      settings: AttributesFormatString=%<Criteria> = %<Threshold>
  P [W] : Outport
  mdotgen [kg/s] : Outport  Port=2
  wires:
  Gain1/1 -> P [W]/1
  Gain/1 -> mdotgen [kg/s]/1
  u [1/0]/1 -> Switch/2
  Switch/1 -> Gain1/1, Gain/1
  Constant/1 -> Switch/1
  Constant1/1 -> Switch/3

== system WZM_QSS_Lib/ThermalManagement/HeatFlowTo ==
  Odot [W] : Inport
  Gain : Gain  Gain=idx
  QdotVec [W] : Outport
  wires:
  Odot [W]/1 -> Gain/1
  Gain/1 -> QdotVec [W]/1

== system WZM_QSS_Lib/ThermalManagement/HeatFlow_VarTemp ==
  mdot [kg/s] : Inport
  Theta_in [K] : Inport  Port=2
  Theta_out [K] : Inport  Port=3
  Gain : Gain  Gain=cp
  Product : Product  RndMeth=Zero
  Subtract : Sum  Inputs=-+
  Qdot [W] : Outport
  wires:
  Gain/1 -> Product/1
  mdot [kg/s]/1 -> Gain/1
  Theta_in [K]/1 -> Subtract/1
  Theta_out [K]/1 -> Subtract/2
  Subtract/1 -> Product/2
  Product/1 -> Qdot [W]/1

== system WZM_QSS_Lib/ThermalManagement/Housing ==
  on [1/0] : Inport
  Qdot_in [W] : Inport  Port=2
  Theta_amb [K] : Inport  Port=3
  Housing_AirCooledFan_ao : WZM_QSS_Lib/ThermalManagement/Housing_AirCooledFan_ao  SystemSampleTime=-1  Cabinet=0  Fan=0
  P_el[W] : Outport
  Qdot [W] : Outport  Port=2
  QdotExtr [W] : Outport  Port=3
  T_Housing [K] : Outport  Port=4
  wires:
  on [1/0]/1 -> Housing_AirCooledFan_ao/1
  Qdot_in [W]/1 -> Housing_AirCooledFan_ao/2
  Theta_amb [K]/1 -> Housing_AirCooledFan_ao/3
  Housing_AirCooledFan_ao/1 -> P_el[W]/1
  Housing_AirCooledFan_ao/2 -> Qdot [W]/1
  Housing_AirCooledFan_ao/3 -> QdotExtr [W]/1
  Housing_AirCooledFan_ao/4 -> T_Housing [K]/1

== system WZM_QSS_Lib/ThermalManagement/Housing_AirCooledFan_ao ==
  on [1/0] : Inport
  Qdot_in [W] : Inport  Port=2
  Theta_amb [K] : Inport  Port=3
  Constant : Constant  Value=0
  Fan : Subsystem  BlockChoice=Fan_OPPoint
      link override Fan_OPPoint: Vdotnom=Fan.Vdotnom  Pnom=Fan.Pnom
      settings: AttributesFormatString=%<BlockChoice>  TemplateBlock=WZM_QSS_Lib/ThermalManagement/Fan  MemberBlocks=Fan_OPPoint,Fan_OPPoint_onoff
  HeatFlow_VarTemp : WZM_QSS_Lib/ThermalManagement/HeatFlow_VarTemp  SystemSampleTime=-1  cp=1005
  Housing : WZM_QSS_Lib/ThermalManagement/Thermal Element  SystemSampleTime=-1  m=Cabinet.m  cp=Cabinet.cp  R=Cabinet.R  A=Cabinet.A
  P_el[W] : Outport
  Qdot [W] : Outport  Port=2
  QdotExtr [W] : Outport  Port=3
  T_Housing [K] : Outport  Port=4
  wires:
  on [1/0]/1 -> Fan/2(u [1/0])
  Constant/1 -> Fan/1(mdot [kg/s])
  Theta_amb [K]/1 -> Housing/3, HeatFlow_VarTemp/2
  Housing/1 -> T_Housing [K]/1, HeatFlow_VarTemp/3
  Fan/1(P [W]) -> P_el[W]/1
  Housing/2 -> Qdot [W]/1
  Fan/2(mdotgen [kg/s]) -> HeatFlow_VarTemp/1
  HeatFlow_VarTemp/1 -> Housing/2, QdotExtr [W]/1
  Qdot_in [W]/1 -> Housing/1

== system WZM_QSS_Lib/ThermalManagement/Housing_Dummy ==
  on [1/0] : Inport
  Qdot_in [W] : Inport  Port=2
  Theta_amb [K] : Inport  Port=3
  Constant : Constant  Value=0
  Constant1 : Constant  Value=0
  Terminator : Terminator
  P_el[W] : Outport
  Qdot [W] : Outport  Port=2
  QdotExtr [W] : Outport  Port=3
  T_Housing [K] : Outport  Port=4
  wires:
  Theta_amb [K]/1 -> T_Housing [K]/1
  Qdot_in [W]/1 -> Qdot [W]/1
  Constant/1 -> QdotExtr [W]/1
  Constant1/1 -> P_el[W]/1
  on [1/0]/1 -> Terminator/1

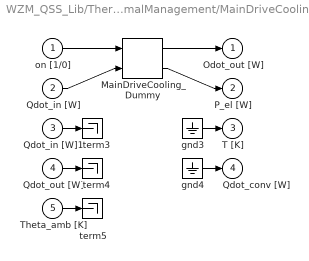
== system WZM_QSS_Lib/ThermalManagement/MainDriveCooling ==
  on [1/0] : Inport
  Qdot_in [W] : Inport  Port=2
  Qdot_in [W]1 : Inport  Port=3
  Qdot_out [W] : Inport  Port=4
  Theta_amb [K] : Inport  Port=5
  MainDriveCooling_Dummy : WZM_QSS_Lib/ThermalManagement/MainDriveCooling_Dummy  SystemSampleTime=-1
  gnd3 : Ground
  gnd4 : Ground
  term3 : Terminator
  term4 : Terminator
  term5 : Terminator
  Odot_out [W] : Outport
  P_el [W] : Outport  Port=2
  T [K] : Outport  Port=3
  Qdot_conv [W] : Outport  Port=4
  wires:
  on [1/0]/1 -> MainDriveCooling_Dummy/1
  Qdot_in [W]/1 -> MainDriveCooling_Dummy/2
  MainDriveCooling_Dummy/1 -> Odot_out [W]/1
  MainDriveCooling_Dummy/2 -> P_el [W]/1
  Qdot_in [W]1/1 -> term3/1
  Qdot_out [W]/1 -> term4/1
  Theta_amb [K]/1 -> term5/1
  gnd3/1 -> T [K]/1
  gnd4/1 -> Qdot_conv [W]/1

== system WZM_QSS_Lib/ThermalManagement/MainDriveCoolingEx ==
  Q_Spindel : Inport
  Theta_amb [K] : Inport  Port=2
  on [1/0] : Inport  Port=3
  AirCooling : Subsystem  mask{epsilon=AirCooling.epsilon, T_int=AirCooling.T_int, T_ext=AirCooling.T_ext, Qdot=AirCooling.Qdot}
      mask prompts: epsilon "Kühlleistung"; T_int "T intern"; T_ext "T extern"; Qdot "KühlleistungAnlage"
  Constant : Constant  Value=0
  Controller : Relay  OnSwitchValue=TController.Tmax  OffSwitchValue=TController.Tmin
  Switch : Switch  Criteria=u2 > Threshold
  Temperatur : Subsystem  mask{m=Temperatur.m, cp=Temperatur.cp, A=Temperatur.A, R=Temperatur.R}
      mask prompts: m "Masse"; cp "Wärmecoefficient"; A "Fläche"; R "Durchgangscoefficient"
  Qdot_Oberflaeche : Outport
  P_el [W] : Outport  Port=2
  Q_Kuehlung : Outport  Port=3
  T_Spindel : Outport  Port=4
  wires:
  Switch/1 -> AirCooling/1(On [1/0])
  Constant/1 -> Switch/3
  on [1/0]/1 -> Switch/2
  Temperatur/2(Qdot_Oberflaeche [W]) -> Qdot_Oberflaeche/1
  AirCooling/1(P_el [W]) -> P_el [W]/1
  AirCooling/2(Q_Kuehlung) -> Temperatur/2(Q_Kuehlung), Q_Kuehlung/1
  Q_Spindel/1 -> Temperatur/1(Q_Spindel)
  Theta_amb [K]/1 -> AirCooling/3(T_ext [K]), Temperatur/3(Theta_amb [K])
  Temperatur/1(T [K]) -> AirCooling/2(T_spuhle [K]), Controller/1, T_Spindel/1
  Controller/1 -> Switch/1

== system WZM_QSS_Lib/ThermalManagement/MainDriveCooling_Dummy ==
  on [1/0] : Inport
  Qdot_in [W] : Inport  Port=2
  Constant : Constant  Value=0
  Terminator : Terminator
  Odot_out [W] : Outport
  P_el [W] : Outport  Port=2
  wires:
  Qdot_in [W]/1 -> Odot_out [W]/1
  Constant/1 -> P_el [W]/1
  on [1/0]/1 -> Terminator/1

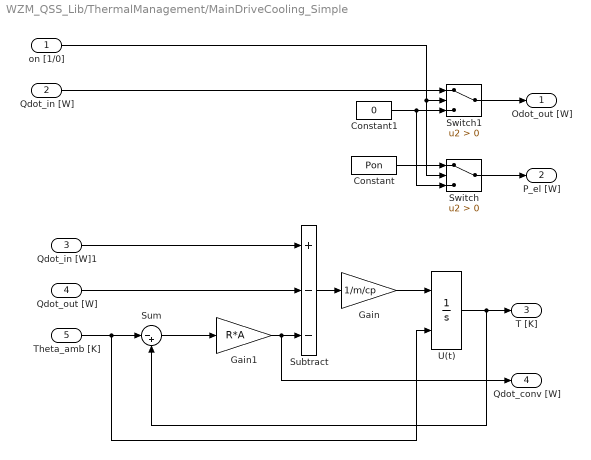
== system WZM_QSS_Lib/ThermalManagement/MainDriveCooling_Simple ==
  on [1/0] : Inport
  Qdot_in [W] : Inport  Port=2
  Qdot_in [W]1 : Inport  Port=3
  Qdot_out [W] : Inport  Port=4
  Theta_amb [K] : Inport  Port=5
  Constant : Constant  Value=Pon
  Constant1 : Constant  Value=0
  Gain : Gain  Gain=1/m/cp
  Gain1 : Gain  Gain=R*A
  Subtract : Sum  Inputs=+--
  Sum : Sum  Inputs=|-+
  Switch : Switch  Criteria=u2 > Threshold
  Switch1 : Switch  Criteria=u2 > Threshold
  U(t) : Integrator  InitialConditionSource=external
  Odot_out [W] : Outport
  P_el [W] : Outport  Port=2
  T [K] : Outport  Port=3
  Qdot_conv [W] : Outport  Port=4
  wires:
  Qdot_in [W]/1 -> Switch1/1
  Constant/1 -> Switch/1
  Switch1/1 -> Odot_out [W]/1
  Switch/1 -> P_el [W]/1
  on [1/0]/1 -> Switch1/2, Switch/2
  Constant1/1 -> Switch1/3, Switch/3
  Gain/1 -> U(t)/1
  Gain1/1 -> Qdot_conv [W]/1, Subtract/3
  Sum/1 -> Gain1/1
  Theta_amb [K]/1 -> U(t)/2, Sum/1
  Subtract/1 -> Gain/1
  Qdot_out [W]/1 -> Subtract/2
  Qdot_in [W]1/1 -> Subtract/1
  U(t)/1 -> Sum/2, T [K]/1

== system WZM_QSS_Lib/ThermalManagement/ProcessCooling ==
  on [1/0] : Inport
  Qdot_in [W] : Inport  Port=2
  ProcessCooling_Dummy : WZM_QSS_Lib/ThermalManagement/ProcessCooling_Dummy  SystemSampleTime=-1
  Odot_out [W] : Outport
  P_el [W] : Outport  Port=2
  mdot_air [m^3/s] : Outport  Port=3
  mdot_cf [m^3/s] : Outport  Port=4
  wires:
  on [1/0]/1 -> ProcessCooling_Dummy/1
  Qdot_in [W]/1 -> ProcessCooling_Dummy/2
  ProcessCooling_Dummy/1 -> Odot_out [W]/1
  ProcessCooling_Dummy/2 -> P_el [W]/1
  ProcessCooling_Dummy/3 -> mdot_air [m^3/s]/1
  ProcessCooling_Dummy/4 -> mdot_cf [m^3/s]/1

== system WZM_QSS_Lib/ThermalManagement/ProcessCooling_Dummy ==
  on [1/0] : Inport
  Qdot_in [W] : Inport  Port=2
  Constant : Constant  Value=0
  Constant1 : Constant  Value=0
  Constant2 : Constant  Value=0
  Terminator : Terminator
  Odot_out [W] : Outport
  P_el [W] : Outport  Port=2
  mdot_air [m^3/s] : Outport  Port=3
  mdot_cf [m^3/s] : Outport  Port=4
  wires:
  on [1/0]/1 -> Terminator/1
  Constant/1 -> P_el [W]/1
  Qdot_in [W]/1 -> Odot_out [W]/1
  Constant1/1 -> mdot_air [m^3/s]/1
  Constant2/1 -> mdot_cf [m^3/s]/1

== system WZM_QSS_Lib/ThermalManagement/ProcessCooling_Simple ==
  on [1/0] : Inport
  Qdot_in [W] : Inport  Port=2
  Constant : Constant  Value=0
  Constant1 : Constant  Value=Pconst
  Constant2 : Constant  Value=0
  Gain : Gain  Gain=1/1005/297
  Saturation : Saturate  UpperLimit=Inf  LowerLimit=0
  Saturation1 : Saturate  UpperLimit=Inf  LowerLimit=0
  Switch : Switch  Criteria=u2 > Threshold
  Switch1 : Switch  Criteria=u2 > Threshold
  Odot_out [W] : Outport
  P_el [W] : Outport  Port=2
  mdot_air [m^3/s] : Outport  Port=3
  wires:
  Qdot_in [W]/1 -> Odot_out [W]/1, Gain/1
  Constant1/1 -> Switch/1
  on [1/0]/1 -> Switch/2, Switch1/2
  Constant/1 -> Switch/3
  Switch/1 -> Saturation1/1
  Switch1/1 -> Saturation/1
  Constant2/1 -> Switch1/3
  Gain/1 -> Switch1/1
  Saturation/1 -> mdot_air [m^3/s]/1
  Saturation1/1 -> P_el [W]/1

== system WZM_QSS_Lib/ThermalManagement/Thermal Element ==
  Qdot_in [W] : Inport
  Qdot_out [W] : Inport  Port=2
  Theta_amb [K] : Inport  Port=3
  Gain : Gain  Gain=1/m/cp
  Gain1 : Gain  Gain=R*A
  Subtract : Sum  Inputs=+--
  Sum : Sum  Inputs=|-+
  U(t) : Integrator  InitialConditionSource=external  ZeroCross=off
  T [K] : Outport
  Qdot_conv [W] : Outport  Port=2
  wires:
  U(t)/1 -> T [K]/1, Sum/2
  Qdot_in [W]/1 -> Subtract/1
  Qdot_out [W]/1 -> Subtract/2
  Subtract/1 -> Gain/1
  Theta_amb [K]/1 -> Sum/1, U(t)/2
  Sum/1 -> Gain1/1
  Gain1/1 -> Subtract/3, Qdot_conv [W]/1
  Gain/1 -> U(t)/1

== system WZM_QSS_Lib/Assembly/Turning Machine/AirCompressor ==
  on [1/0] : Inport
  mdot [kg/s] : Inport  Port=2
  AirCompressor_Simple : WZM_QSS_Lib/AirSystem/AirCompressor_Simple  SystemSampleTime=-1  Pstandby=AirCompressor.Pstandby  Pworking=AirCompressor.Pworking
  gnd2 : Ground
  P_el [W] : Outport
  Qdot [W] : Outport  Port=2
  wires:
  on [1/0]/1 -> AirCompressor_Simple/1
  mdot [kg/s]/1 -> AirCompressor_Simple/2
  AirCompressor_Simple/1 -> P_el [W]/1
  gnd2/1 -> Qdot [W]/1

== system WZM_QSS_Lib/Assembly/Turning Machine/CNC_Cabinet ==
  on [1/0] : Inport
  P_SimDrv [W] : Inport  Port=2
  P_el [W] : Inport  Port=3
  Theta_amb [K] : Inport  Port=4
  CNC_Cabinet_AirAirCooled_Hyst : WZM_QSS_Lib/Electronics/CNC_Cabinet_AirAirCooled_Hyst  SystemSampleTime=-1  Cabinet=CNC.Cabinet  Cooling=CNC.Cooling  SimoDrive=CNC.SimoDrive
  P_eltot [W] : Outport
  P_CNC [W] : Outport  Port=2
  P_Cooling [W] : Outport  Port=3
  Qdot [W] : Outport  Port=4
  QdotExtr [W] : Outport  Port=5
  T_CNC [K] : Outport  Port=6
  wires:
  on [1/0]/1 -> CNC_Cabinet_AirAirCooled_Hyst/1
  P_SimDrv [W]/1 -> CNC_Cabinet_AirAirCooled_Hyst/2
  P_el [W]/1 -> CNC_Cabinet_AirAirCooled_Hyst/3
  Theta_amb [K]/1 -> CNC_Cabinet_AirAirCooled_Hyst/4
  CNC_Cabinet_AirAirCooled_Hyst/1 -> P_eltot [W]/1
  CNC_Cabinet_AirAirCooled_Hyst/2 -> P_CNC [W]/1
  CNC_Cabinet_AirAirCooled_Hyst/3 -> P_Cooling [W]/1
  CNC_Cabinet_AirAirCooled_Hyst/4 -> Qdot [W]/1
  CNC_Cabinet_AirAirCooled_Hyst/5 -> QdotExtr [W]/1
  CNC_Cabinet_AirAirCooled_Hyst/6 -> T_CNC [K]/1

== system WZM_QSS_Lib/Assembly/Turning Machine/Housing ==
  on [1/0] : Inport
  Qdot_in [W] : Inport  Port=2
  Theta_amb [K] : Inport  Port=3
  Housing_AirCooledFan_ao : WZM_QSS_Lib/ThermalManagement/Housing_AirCooledFan_ao  SystemSampleTime=-1  Cabinet=Housing.Cabinet  Fan=Housing.Fan
  P_el[W] : Outport
  Qdot [W] : Outport  Port=2
  QdotExtr [W] : Outport  Port=3
  T_Housing [K] : Outport  Port=4
  wires:
  on [1/0]/1 -> Housing_AirCooledFan_ao/1
  Qdot_in [W]/1 -> Housing_AirCooledFan_ao/2
  Theta_amb [K]/1 -> Housing_AirCooledFan_ao/3
  Housing_AirCooledFan_ao/1 -> P_el[W]/1
  Housing_AirCooledFan_ao/2 -> Qdot [W]/1
  Housing_AirCooledFan_ao/3 -> QdotExtr [W]/1
  Housing_AirCooledFan_ao/4 -> T_Housing [K]/1

== system WZM_QSS_Lib/Assembly/Turning Machine/HydraulicPump ==
  on [1/0] : Inport
  P_hyd [W] : Inport  Port=2
  HydraulicPump_Simple : WZM_QSS_Lib/Hydraulics/HydraulicPump_Simple  SystemSampleTime=-1  Pconst=HydraulicPump.Pconst
  P_el [W] : Outport
  Qdot [W] : Outport  Port=2
  wires:
  on [1/0]/1 -> HydraulicPump_Simple/1
  P_hyd [W]/1 -> HydraulicPump_Simple/2
  HydraulicPump_Simple/1 -> P_el [W]/1
  HydraulicPump_Simple/2 -> Qdot [W]/1

== system WZM_QSS_Lib/Assembly/Turning Machine/MainDrive ==
  on [1/0] : Inport
  omega_dem [rad/s] : Inport  Port=2
  M_dem [Nm] : Inport  Port=3
  MainDrive_simple : WZM_QSS_Lib/Drives/MainDrive_simple  SystemSampleTime=-1  P_max=MainDrive.Pmax  eta=MainDrive.eta  theta=MainDrive.Theta  Tomega=MainDrive.Tabelomega  TM=MainDrive.TabelM  Teta=MainDrive.Tabeleta
  gnd3 : Ground
  gnd5 : Ground
  term1 : Terminator
  P_mech [W] : Outport
  P_el [W] : Outport  Port=2
  P_hyd [W] : Outport  Port=3
  Q_dot [W] : Outport  Port=4
  mdot_air [m^3/s] : Outport  Port=5
  n MainDrive : Outport  Port=6
  wires:
  omega_dem [rad/s]/1 -> MainDrive_simple/1
  M_dem [Nm]/1 -> MainDrive_simple/2
  MainDrive_simple/1 -> P_mech [W]/1
  MainDrive_simple/2 -> Q_dot [W]/1
  MainDrive_simple/3 -> P_el [W]/1
  MainDrive_simple/4 -> n MainDrive/1
  on [1/0]/1 -> term1/1
  gnd3/1 -> P_hyd [W]/1
  gnd5/1 -> mdot_air [m^3/s]/1

== system WZM_QSS_Lib/Assembly/Turning Machine/ProcessCooling ==
  on [1/0] : Inport
  Qdot_in [W] : Inport  Port=2
  ProcessCooling_Simple : WZM_QSS_Lib/ThermalManagement/ProcessCooling_Simple  SystemSampleTime=-1  Pconst=ProcessCooling.Pconst
  gnd4 : Ground
  Odot_out [W] : Outport
  P_el [W] : Outport  Port=2
  mdot_air [m^3/s] : Outport  Port=3
  mdot_cf [m^3/s] : Outport  Port=4
  wires:
  on [1/0]/1 -> ProcessCooling_Simple/1
  Qdot_in [W]/1 -> ProcessCooling_Simple/2
  ProcessCooling_Simple/1 -> Odot_out [W]/1
  ProcessCooling_Simple/2 -> P_el [W]/1
  ProcessCooling_Simple/3 -> mdot_air [m^3/s]/1
  gnd4/1 -> mdot_cf [m^3/s]/1

== system WZM_QSS_Lib/Assembly/Turning Machine/ProcessModel ==
  P_mech : Inport
  Process_simple : WZM_QSS_Lib/Process/Process_simple  SystemSampleTime=-1  eta=Process.eta
  gnd2 : Ground
  Odot [W] : Outport
  mdot_waste [kg/s] : Outport  Port=2
  wires:
  P_mech/1 -> Process_simple/1
  Process_simple/1 -> Odot [W]/1
  gnd2/1 -> mdot_waste [kg/s]/1

== system WZM_QSS_Lib/Drives/MainDrive_simple/Controller ==
  e [rad/s] : Inport
  T_dem [Nm] : Inport  Port=2
  Gin3 : Gain  Gain=theta*0.5
  Subtract1 : Sum
  T_u : Outport
  wires:
  Subtract1/1 -> T_u/1  "T(t)"
  Gin3/1 -> Subtract1/1
  T_dem [Nm]/1 -> Subtract1/2
  e [rad/s]/1 -> Gin3/1

== system WZM_QSS_Lib/Drives/MainDrive_simple/Power saturation ==
  omega [rad/s] : Inport
  T [Nm] : Inport  Port=2
  Divide : Product  Inputs=*/
  Product1 : Product  RndMeth=Zero
  Saturation : Saturate  UpperLimit=P_max  LowerLimit=-P_max
  Switch : Switch  Criteria=u2 ~= 0
  T_sat [Nm] : Outport
  wires:
  Product1/1 -> Saturation/1
  T [Nm]/1 -> Product1/1, Switch/3
  omega [rad/s]/1 -> Product1/2, Divide/2, Switch/2
  Saturation/1 -> Divide/1
  Divide/1 -> Switch/1
  Switch/1 -> T_sat [Nm]/1

== system WZM_QSS_Lib/Electronics/CNC_Cabinet_AirCooledFan_ao/Fan ==
  mdot [kg/s] : Inport
  u [1/0] : Inport  Port=2
  Fan_OPPoint_onoff : WZM_QSS_Lib/ThermalManagement/Fan_OPPoint_onoff  SystemSampleTime=-1  Vdotnom=1  Pnom=1  rho=1.2
      settings: AttributesFormatString=Vdotnom = %<Vdotnom> m^3/s\nPnom = %<Pnom> W\nDesity = %<rho> kg/m^3
  term1 : Terminator
  P [W] : Outport
  mdotgen [kg/s] : Outport  Port=2
  wires:
  u [1/0]/1 -> Fan_OPPoint_onoff/1
  Fan_OPPoint_onoff/1 -> P [W]/1
  Fan_OPPoint_onoff/2 -> mdotgen [kg/s]/1
  mdot [kg/s]/1 -> term1/1

== system WZM_QSS_Lib/ThermalManagement/Housing_AirCooledFan_ao/Fan ==
  mdot [kg/s] : Inport
  u [1/0] : Inport  Port=2
  Fan_OPPoint : WZM_QSS_Lib/ThermalManagement/Fan_OPPoint  SystemSampleTime=-1  Vdotnom=Fan.Vdotnom  Pnom=Fan.Pnom  rho=1.2
      settings: AttributesFormatString=Vdotnom = %<Vdotnom> m^3/s\nPnom = %<Pnom> W\nDesity = %<rho> kg/m^3
  term2 : Terminator
  P [W] : Outport
  mdotgen [kg/s] : Outport  Port=2
  wires:
  mdot [kg/s]/1 -> Fan_OPPoint/1
  Fan_OPPoint/1 -> P [W]/1
  Fan_OPPoint/2 -> mdotgen [kg/s]/1
  u [1/0]/1 -> term2/1

== system WZM_QSS_Lib/ThermalManagement/MainDriveCoolingEx/AirCooling ==
  On [1/0] : Inport
  T_spuhle [K] : Inport  Port=2
  T_ext [K] : Inport  Port=3
  Constant : Constant  Value=0
  Gain : Gain  Gain=1/epsilon
  Lookup Table (n-D) : Lookup_n-D  BreakpointsForDimension1=T_int  BreakpointsForDimension2=T_ext  Table=Qdot  InterpMethod=Cubic spline  InputSameDT=on
  Saturation : Saturate  UpperLimit=4000  LowerLimit=2000
  Switch : Switch  Criteria=u2 > Threshold
  P_el [W] : Outport
  Q_Kuehlung : Outport  Port=2
  wires:
  T_ext [K]/1 -> Lookup Table (n-D)/2
  T_spuhle [K]/1 -> Lookup Table (n-D)/1
  On [1/0]/1 -> Switch/2
  Constant/1 -> Switch/3
  Switch/1 -> Gain/1, Q_Kuehlung/1
  Gain/1 -> P_el [W]/1
  Saturation/1 -> Switch/1
  Lookup Table (n-D)/1 -> Saturation/1
